simulink model "Simulink_MotorCC"  (R2024a)
settings: Solver=VariableStepAuto  StartTime=0.0  StopTime=35  RelTol=1e-3
values from neighbouring files (symbols this model uses):
  den = [2.7 3.36 0.53]    [Projeto_MalhaAberta.m]    (also in Projeto_MotorCC.m)
  num = 4.2    [Projeto_MalhaAberta.m]    (also in Projeto_MotorCC.m)
undefined symbols (not defined in the file or in its folder): Kd, Ki, Kp
settings Model: LastModifiedBy=daniel

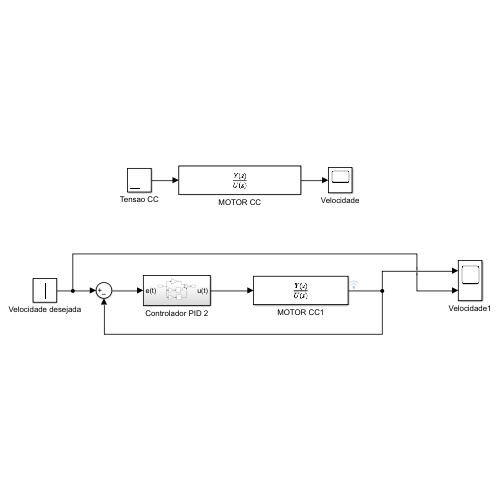
[thumbnail: Simulink's stored preview of the top-level diagram]
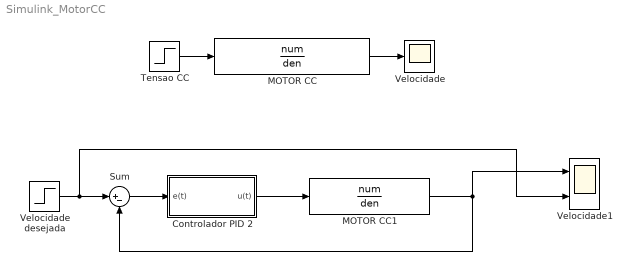
== system Simulink_MotorCC ==
  Controlador PID 2 : Subsystem
  MOTOR CC : TransferFcn  Numerator=num  Denominator=den
  MOTOR CC1 : TransferFcn  Numerator=num  Denominator=den
  Sum : Sum  Inputs=|+-
  Tensao CC : Step  After=5  SampleTime=0
  Velocidade : Scope
  Velocidade desejada : Step  SampleTime=0
  Velocidade1 : Scope  NumInputPorts=2
  wires:
  Tensao CC/1 -> MOTOR CC/1
  MOTOR CC/1 -> Velocidade/1
  MOTOR CC1/1 -> Sum/2, Velocidade1/1
  Velocidade desejada/1 -> Velocidade1/2, Sum/1
  Sum/1 -> Controlador PID 2/1(e(t))
  Controlador PID 2/1(u(t)) -> MOTOR CC1/1

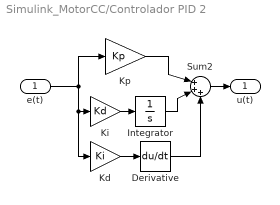
== system Simulink_MotorCC/Controlador PID 2 ==
  e(t) : Inport
  Derivative : Derivative
  Integrator : Integrator
  Kd : Gain  Gain=Ki
  Ki : Gain  Gain=Kd
  Kp : Gain  Gain=Kp
  Sum2 : Sum  Inputs=|+++
  u(t) : Outport
  wires:
  e(t)/1 -> Kd/1, Ki/1, Kp/1
  Derivative/1 -> Sum2/3
  Kd/1 -> Derivative/1
  Kp/1 -> Sum2/1
  Ki/1 -> Integrator/1
  Integrator/1 -> Sum2/2
  Sum2/1 -> u(t)/1
